simulink model "PowerOut_EmulatedPanel_ST"  (R2018b)
settings: Solver=ode23tb  StartTime=0.0  StopTime=20  MaxStep=0.1  RelTol=1e-4  EnableMultiTasking=on
PreLoadFcn:
  | Ts = 1e-6;
  | G = 1000;
  | PVCellIsc = 7;
  | PVCellVoc = 0.64;
  | PVCellRs = 0.001;
  | tau = 1e-4;
  | 
  | load EmulatedPV_Data.mat;
InitFcn:
  | ArrayPower = ArrayCurrent.*ArrayVoltage;
values from neighbouring files (symbols this model uses):
  ArrayCurrent = [3 2.95271067684 2.90135967378 2.84545649231 2.78442846347 2.71757715417 2.64406556825 2.56286559221 2.47269969012 2.37192388363 2.25842875672 2.12940283602 ... (900 elements, 100x9)]    [EmulatedPV_Data.mat]
  ArrayVoltage = [0 0.30303030303 0.606060606061 0.909090909091 1.21212121212 1.51515151515 1.81818181818 2.12121212121 2.42424242424 2.72727272727 3.0303030303 3.33333333333 ... (100 elements, 100x1)]    [EmulatedPV_Data.mat]
  Irradiance = [0.2 0.3 0.4 0.5 0.6 0.7 0.8 0.9 1]    [EmulatedPV_Data.mat]
libraries: powerlib x6, simulink x3, simulink_extras x1
settings Model: Creator=cosorio  LastModifiedBy=jlesage
settings DataIOCC: SaveFormat=Array  SignalLoggingSaveFormat=ModelDataLogs  SaveOutput=off  DSMLogging=off  SaveTime=off  OutputTimes=[0]
settings OptimizationCC: ExpressionDepthLimit=2147483647  LifeSpan=inf
settings DebuggingCC: UnderspecifiedInitializationDetection=Classic  MergeDetectMultiDrivingBlocksExec=none  SolverPrmCheckMsg=warning  FcnCallInpInsideContextMsg=warning  AllowSymbolicDim=off  StateNameClashWarn=warning  LibraryContextMissingDiagnostic=none  SFUnexpectedBacktrackingDiag=warning  SFNoUnconditionalDefaultTransitionDiag=warning  SFExecutionAtInitializationDiag=none
settings HardwareCC: ProdBitPerPointer=32  ProdBitPerSizeT=32  ProdBitPerPtrDiffT=32  ProdLargestAtomicFloat=None  ProdIntDivRoundTo=Undefined  ProdEndianess=Unspecified  ProdWordSize=32  ProdHWDeviceType=32-bit Generic
settings ModelReferenceCC: PropagateSignalLabelsOutOfModel=off
settings SFSimCC: SimUseLocalCustomCode=off
settings RTWCC: RTWUseLocalCustomCode=off
settings CodeAppCC: StateflowObjectComments=on
settings GRTTargetCC: TargetLangStandard=C89/C90 (ANSI)  GeneratePreprocessorConditionals=Disable all  CombineOutputUpdateFcns=off  GRTInterface=on
settings ConfigComp: CovMetricSettings=dw  CovHtmlReporting=on  CovSaveCumulativeToWorkspaceVar=on  CovSaveSingleToWorkspaceVar=on  CovExternalEMLEnable=off  CovSFcnEnable=off
settings SimscapeCC: SimscapeNormalizeSystem=off

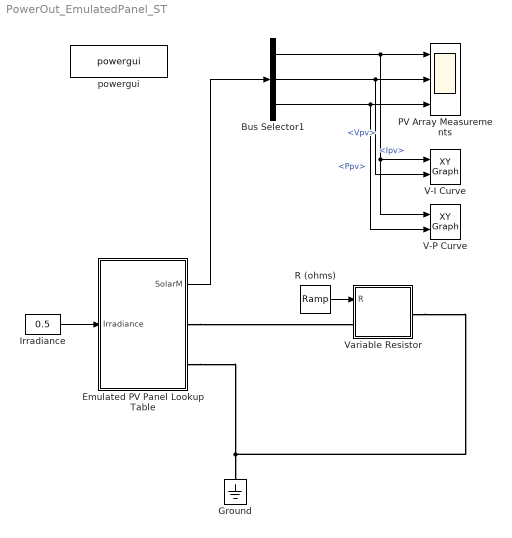
== system PowerOut_EmulatedPanel_ST ==
  Bus Selector1 : BusSelector  OutputSignals=Vpv,Ipv,Ppv
  Emulated PV Panel Lookup Table : Subsystem
      mask Display:
      | image(imread('panel.jpg'))
      | color('yellow')
      | port_label('input',1,'Ir')
      | port_label('output',1,'m')
      | port_label('Rconn',1,'A')
      | port_label('Rconn',2,'B')
  Ground : powerlib/Elements/Ground  LConnTagsString=a
      settings: SourceProductName=Simscape Electrical
  Irradiance : Constant  Value=0.5  OutDataTypeStr=double
  PV Array Measurements : Scope  NumInputPorts=3
  R (ohms) : simulink/Sources/Ramp  slope=2  start=0  InitialOutput=0
  V-I Curve : simulink/Sinks/XY Graph  xmin=0  xmax=30  ymin=0  ymax=3  st=-1
  V-P Curve : simulink/Sinks/XY Graph  xmin=0  xmax=30  ymin=0  ymax=40  st=-1
  Variable Resistor : Subsystem  mask(Variable Resistor){Isc=2*PVCellIsc*G/1000, tau=tau}
      mask prompts: Isc "Initial Output Current (A) :"; tau "Time constant (sec):"
      mask help:
      | Simulink implementation of a variable resistor.
      |
      | A first order transfer function is used to break the algebraic loop. The time constant of this transfer function should be adjusted such that it will not significantly affect the model dynamics.
  powergui : powerlib/powergui  Priority=1  SimulationMode=Continuous  SampleTime=Ts  frequency=60  Iterations=50  frequencyindice=0  Pbase=100e6  ErrMax=1e-4  UnitsV=kV  UnitsW=MW  buscounter=0  FunctionMessages=off  echomessages=off  EnableUseOfTLC=off  CurrentSourceSwitches=on  DisableSnubberDevices=off  DisableRonSwitches=off  DisableVfSwitches=off  DisplayEquations=off  SolverType=Tustin  Interpol=off  ExternalGateDelay=off  methode=off  Ts=0  x0status=blocks  SPID=off  SwTol=0  HookPort=off  RestoreLinks=warning  ResistiveCurrentMeasurement=off  Frange=[0:2:500]  Ylog=off  Xlog=on  ShowGrid=off  save=off  variable=ZData  structure=inverterdata  ZoomFFT=off  StartTime=0.2  cycles=2  DisplayStyle=1  fundamental=60  FreqAxis=on  MaxFrequency=1000  frequencyindicesteady=1  RmsSteady=1  display=off
      settings: SourceProductName=Simscape Electrical
  wires:
  Emulated PV Panel Lookup Table/1(SolarM) -> Bus Selector1/1
  Bus Selector1/1 -> PV Array Measurements/1, V-I Curve/1, V-P Curve/1  "<Vpv>"
  Bus Selector1/2 -> PV Array Measurements/2, V-I Curve/2  "<Ipv>"
  Bus Selector1/3 -> PV Array Measurements/3, V-P Curve/2  "<Ppv>"
  R (ohms)/1 -> Variable Resistor/1(R)
  Irradiance/1 -> Emulated PV Panel Lookup Table/1(Irradiance)
  connections:
  Variable Resistor/RConn1 -- Emulated PV Panel Lookup Table/RConn2 -- Ground/LConn1
  Emulated PV Panel Lookup Table/RConn1 -- Variable Resistor/LConn1

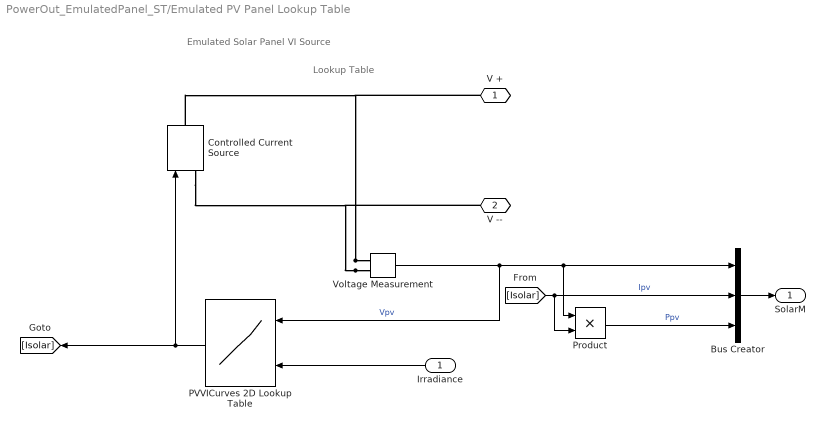
== system PowerOut_EmulatedPanel_ST/Emulated PV Panel Lookup Table ==
  note: Lookup Table
  note: Emulated Solar Panel VI Source
  Irradiance : Inport
  Bus Creator : BusCreator  Inputs=3
  Controlled Current Source : powerlib/Electrical Sources/Controlled Current Source  Initialize=on  Source_Type=AC  Amplitude=0  Phase=0  Frequency=0  Measurements=None
      settings: SourceProductName=Simscape Electrical
  PVVICurves 2D Lookup Table : Lookup_n-D  BreakpointsForDimension1=ArrayVoltage  BreakpointsForDimension2=Irradiance  Table=ArrayCurrent  InternalRulePriority=Speed  RndMeth=Simplest  InputSameDT=on
  Product : Product
  Voltage Measurement : powerlib/Measurements/Voltage Measurement  PhasorSimulation=off  OutputType=Complex  PSBequivalent=0
      settings: SourceProductName=Simscape Electrical
  V + : PMIOPort  Side=Right
  V -- : PMIOPort  Port=2  Side=Right
  SolarM : Outport
  wires:
  Irradiance/1 -> PVVICurves 2D Lookup Table/2
  Bus Creator/1 -> SolarM/1
  Product/1 -> Bus Creator/3  "Ppv"
  PVVICurves 2D Lookup Table/1 -> [Isolar], Controlled Current Source/1
  Voltage Measurement/1 -> Bus Creator/1, Product/1, PVVICurves 2D Lookup Table/1  "Vpv"
  [Isolar] -> Bus Creator/2, Product/2  "Ipv"
  connections:
  Voltage Measurement/LConn2 -- Controlled Current Source/LConn1 -- V --/RConn1
  Voltage Measurement/LConn1 -- Controlled Current Source/RConn1 -- V +/RConn1

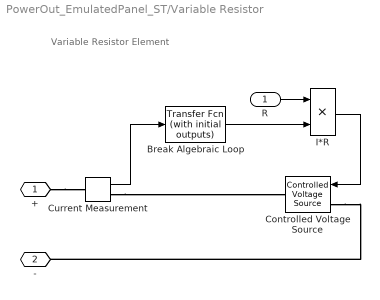
== system PowerOut_EmulatedPanel_ST/Variable Resistor ==
  note: Variable Resistor Element
  R : Inport
  Break Algebraic Loop : simulink_extras/Additional Linear/Transfer Fcn (with initial outputs)  N=[1]  D="[tau  1]"  Y0=Isc  U0=0
  Controlled Voltage Source : powerlib/Electrical Sources/Controlled Voltage Source  Initialize=on  Source_Type=DC  Amplitude=0  Phase=0  Frequency=0  Measurements=None
      settings: SourceProductName=Simscape Electrical
  Current Measurement : powerlib/Measurements/Current Measurement  PhasorSimulation=off  OutputType=Complex  PSBequivalent=0
      settings: SourceProductName=Simscape Electrical
  I*R : Product  Inputs=**
  + : PMIOPort  Side=Left
  - : PMIOPort  Port=2  Side=Right
  wires:
  R/1 -> I*R/1
  Break Algebraic Loop/1 -> I*R/2
  Current Measurement/1 -> Break Algebraic Loop/1
  I*R/1 -> Controlled Voltage Source/1
  connections:
  Controlled Voltage Source/LConn1 -- -/RConn1
  +/RConn1 -- Current Measurement/LConn1
  Current Measurement/RConn1 -- Controlled Voltage Source/RConn1
